simulink model "TBRe19_ECU_SequentialTests"  (R2017b)
settings: Solver=FixedStepDiscrete  StartTime=0.0  StopTime=inf  FixedStep=0.0001  RelTol=1e-3
PostLoadFcn:
  | model_init();
libraries: simulink x28
(part 13 of 22)

== system TBRe19_ECU_SequentialTests/RTDandStateMachine/Pre_Processing_Layer/Pedal_Box ==
  note: Throttle 20 and Brake 10 are arbitrary values (not rules)
  note: Overall Functionality:
      | - All pedal box sensor values are checked to ensure that they are in the correct voltage range
      | - These sensors are then scaled to be between 0-100 %
      | - APPS Implausibility is performed
      | - Brake pedal implausibility is performed
      | - Thresholds for when brake is considered active, and throttle is considered active are set here (used for RTD and Brake Light activation respectively)
  DAL_In : Inport
  APPS and BP Plausibility : Subsystem
  APPS_Implausibility_Check : Subsystem
  BPPS_Implausibility_Check : Subsystem
  Bus Creator : BusCreator  Inputs=12
  Bus Selector : BusSelector  OutputSignals=HAL_Hardwired.Throttle1_Voltage,HAL_Hardwired.Throttle2_Voltage,HAL_Hardwired.Brake_POT,HAL_Hardwired.Brake1_Pressure,HAL_Hardwired.Brake2_Pressure
  Relational Operator : RelationalOperator  OutDataTypeStr=boolean  RndMeth=Simplest
  Relational Operator1 : RelationalOperator  OutDataTypeStr=boolean  RndMeth=Simplest
  Sensor Plausibility : Subsystem
  Terminator : Terminator
  UsbRx : S-Function  FunctionName=NsiUsb_Rx  Parameters=signame,sigtype,resolution,offset,unite,value,is_trigger  SFunctionDeploymentMode=off  EnableBusSupport=off  mask(MUXlink Usb Rx){signame=Brake_Light_Active_Threshold, sigtype=Unsigned Byte, resolution=1, offset=0, unite=%, value=10, is_trigger=off}
      mask prompts: signame "Signal name :"; sigtype "Signal type :"; resolution "Resolution :"; offset "Offset :"; unite "Unit :"; value "Default value :"; is_trigger "Is trigger ?"
      mask help: Receive a frame on the USB Channel.
      mask init:
      | NsiUsb_Rx_InitializationFcn();
      settings: OpenFcn=NsiUsb_Rx_OpenFcn();
      mask Help:
      | eval('block=get_param(gcb, ''RTWdata'');')
      | web([docroot '\toolbox\MUXlink\html\blocks/' block.MUXlink_BlockType '.html'])
      mask Callback signame: NsiUsb_Rx_ApplyFcn(1);
      mask TypeOptions sigtype: Boolean | Signed Byte | Unsigned Byte | Signed Word | Unsigned Word | Signed Double Word | Unsigned Double Word | Single Float | Double Float
      mask Callback sigtype: NsiUsb_Rx_ApplyFcn(2);
      mask Callback resolution: NsiUsb_Rx_ApplyFcn(3);
      mask Callback offset: NsiUsb_Rx_ApplyFcn(4);
      mask Callback unite: NsiUsb_Rx_ApplyFcn(5);
      mask Callback value: NsiUsb_Rx_ApplyFcn(6);
      mask Callback is_trigger: NsiUsb_Rx_ApplyFcn(7);
      mask Display: image(imread('nsi.bmp'));text(0.5, 0.2, 'USB Rx', 'horizontalAlignment', 'center', 'verticalAlignment', 'base');plot([0.05 0.05 0.05 0.05 0.05 0.05 0.05 0.05 0.05 0.05]);port_label('output',1, 'Brake_Light_Active_Threshold');
  UsbRx1 : S-Function  FunctionName=NsiUsb_Rx  Parameters=signame,sigtype,resolution,offset,unite,value,is_trigger  SFunctionDeploymentMode=off  EnableBusSupport=off  mask(MUXlink Usb Rx){signame=Throttle_Active_Threshold, sigtype=Unsigned Byte, resolution=1, offset=0, unite=%, value=5, is_trigger=off}
      mask prompts: signame "Signal name :"; sigtype "Signal type :"; resolution "Resolution :"; offset "Offset :"; unite "Unit :"; value "Default value :"; is_trigger "Is trigger ?"
      mask help: Receive a frame on the USB Channel.
      mask init:
      | NsiUsb_Rx_InitializationFcn();
      settings: OpenFcn=NsiUsb_Rx_OpenFcn();
      mask Help:
      | eval('block=get_param(gcb, ''RTWdata'');')
      | web([docroot '\toolbox\MUXlink\html\blocks/' block.MUXlink_BlockType '.html'])
      mask Callback signame: NsiUsb_Rx_ApplyFcn(1);
      mask TypeOptions sigtype: Boolean | Signed Byte | Unsigned Byte | Signed Word | Unsigned Word | Signed Double Word | Unsigned Double Word | Single Float | Double Float
      mask Callback sigtype: NsiUsb_Rx_ApplyFcn(2);
      mask Callback resolution: NsiUsb_Rx_ApplyFcn(3);
      mask Callback offset: NsiUsb_Rx_ApplyFcn(4);
      mask Callback unite: NsiUsb_Rx_ApplyFcn(5);
      mask Callback value: NsiUsb_Rx_ApplyFcn(6);
      mask Callback is_trigger: NsiUsb_Rx_ApplyFcn(7);
      mask Display: image(imread('nsi.bmp'));text(0.5, 0.2, 'USB Rx', 'horizontalAlignment', 'center', 'verticalAlignment', 'base');plot([0.05 0.05 0.05 0.05 0.05 0.05 0.05 0.05 0.05 0.05]);port_label('output',1, 'Throttle_Active_Threshold');
  Voltage_to_% Conversion : Subsystem
  Pedal_Box_Data : Outport
  wires:
  Bus Creator/1 -> Pedal_Box_Data/1
  DAL_In/1 -> Bus Selector/1
  Voltage_to_% Conversion/1(T1%) -> Bus Creator/2, APPS_Implausibility_Check/1(Throttle1_Per)  "Throttle1_Per"
  Voltage_to_% Conversion/2(T2%) -> Bus Creator/3, APPS_Implausibility_Check/2(Throttle2_Per)  "Throttle2_Per"
  Relational Operator1/1 -> Bus Creator/6  "Throttle_Bool"
  Relational Operator/1 -> Bus Creator/8  "Brake_Bool"
  APPS and BP Plausibility/1(Throttle_%) -> Relational Operator1/1, Bus Creator/5  "Throttle_Percentage"
  APPS and BP Plausibility/2(APPS_BP_Implausibility) -> Bus Creator/7  "APPS_BP_Implausibility"
  APPS_Implausibility_Check/1(APPS_Implausibility) -> Bus Creator/4  "APPS_Implausibility"
  APPS_Implausibility_Check/2(Throttle_%) -> APPS and BP Plausibility/1(Throttle_In)
  Sensor Plausibility/1(Pedal_Sensor_Fail) -> Bus Creator/1  "Pedal_Sensor_Fail"
  Bus Selector/1 -> Sensor Plausibility/1(<Throttle1_Voltage>)  "<Throttle1_Voltage>"
  Bus Selector/2 -> Sensor Plausibility/2(<Throttle2_Voltage>)  "<Throttle2_Voltage>"
  Bus Selector/3 -> Sensor Plausibility/3(<Brake_Voltage>)  "<Brake_POT>"
  Sensor Plausibility/2(TV1_Out) -> Voltage_to_% Conversion/1(Throttle1)
  Sensor Plausibility/3(TV2_Out) -> Voltage_to_% Conversion/2(Throttle2)
  Sensor Plausibility/4(BVPot_Out) -> Voltage_to_% Conversion/3(BrakePOT)
  Bus Selector/4 -> Sensor Plausibility/4(<Brake_Voltage>1)  "<Brake1_Pressure>"
  Bus Selector/5 -> Sensor Plausibility/5(<Brake_Voltage>2)  "<Brake2_Pressure>"
  Sensor Plausibility/5(BV1_Out) -> Voltage_to_% Conversion/4(BrakePress1)
  Sensor Plausibility/6(BV1_Out1) -> Voltage_to_% Conversion/5(BrakePress2)
  BPPS_Implausibility_Check/1(Brake_%) -> Relational Operator/1, Bus Creator/9, APPS and BP Plausibility/2(Brake_%)  "Brake_Percentage"
  BPPS_Implausibility_Check/2(BPPS_Implausibility) -> Bus Creator/10  "BPPS_Implausibility"
  Voltage_to_% Conversion/4(BPr%1) -> Bus Creator/11, BPPS_Implausibility_Check/1(Brake1_Per)  "Brake1_Per"
  Voltage_to_% Conversion/5(BPr%2) -> Bus Creator/12, BPPS_Implausibility_Check/2(Brake2_Per)  "Brake2_Per"
  Voltage_to_% Conversion/3(BPot%) -> Terminator/1  "Brake_%"
  UsbRx/1 -> Relational Operator/2
  UsbRx1/1 -> Relational Operator1/2

== system TBRe19_ECU_SequentialTests/RTDandStateMachine/Vehicle_Functionality_Layer/Vehicle_Operation_Mode ==
  note: Input is zero if error present
  note: NOTE: Check if debounce is needed when coming out of RTD
  note: btnRTD is detected on rising edge
  PrePL_Data : Inport
  Bus Creator : BusCreator  Inputs=5
  Bus Selector1 : BusSelector  OutputSignals=Pedal_Box_Data.Throttle_Bool,Pedal_Box_Data.Brake_Bool,HAL_Data.HAL_Hardwired.btnRTD_Input
  Compare To Constant2 : simulink/Logic and Bit Operations/Compare To Constant  relop=~=  const=0  OutDataTypeStr=boolean
  Operaton_Mode : Stateflow chart  TreatAsAtomicUnit=on
  Rising Edge Detector : Logic  AllPortsSameDT=off  OutDataTypeStr=boolean
  System_Error : Subsystem
  TSS : Subsystem
  Threshold_Level1 : Constant  Value=true  OutDataTypeStr=boolean
  WasZero : Logic  Operator=NOT  AllPortsSameDT=off  OutDataTypeStr=boolean
  prvP2S : Delay  DelayLength=1  InitialCondition=0
  VOM_Data : Outport
  wires:
  Bus Selector1/2 -> Operaton_Mode/2(Brake)  "<Brake_Bool>"
  Compare To Constant2/1 -> Bus Creator/4  "ECU_Ok"
  System_Error/1(System_Error) -> Operaton_Mode/5(Error)
  Operaton_Mode/2(Control_Word) -> Bus Creator/2  "Control_Word"
  Operaton_Mode/1(MCU_NMT_Mode) -> Bus Creator/1  "MCU_NMT_Mode"
  Operaton_Mode/3(State) -> Bus Creator/3, Compare To Constant2/1  "Operation_Mode"
  Bus Creator/1 -> VOM_Data/1  "Vehicle_Operation_Data"
  Bus Selector1/1 -> Operaton_Mode/1(Throttle)  "<Throttle_Bool>"
  PrePL_Data/1 -> Bus Selector1/1, System_Error/1(Errors), TSS/1(PrePL_Data)
  Threshold_Level1/1 -> Operaton_Mode/6(TSS), Bus Creator/5  "TSS"
  WasZero/1 -> Rising Edge Detector/2
  prvP2S/1 -> WasZero/1
  Rising Edge Detector/1 -> Operaton_Mode/3(btnRTD)  "RTD"
  Bus Selector1/3 -> Operaton_Mode/4(btnRTD_Hold), prvP2S/1, Rising Edge Detector/1  "<btnRTD_Input>"

== system TBRe19_ECU_SequentialTests/TSS/Comms_And_Data_Acquisition_Layer/BMS_CAN ==
  note: Overall Functionality:
      | Read CAN messages related to BMS
  Bus Creator4 : BusCreator  Inputs=9
  CanRx6 : S-Function  FunctionName=NsiCan_Rx_Ext  Parameters=data_can,channel,msg_name,ident,ident_type,dlc,signals,is_trigger,is_physical,is_canfd,is_rxgw  SFunctionDeploymentMode=off  EnableBusSupport=off  mask(MUXlink Can Rx){data_can=1;HIGH_SPEED;500Kbps;120 Ohm;C:\Users\TBRe-admin\Documents\Database\TBRe19_DBC_190517.dbc;0;;;0;HIGH_SPEED;500Kbps;120 Ohm;C:\Users\TBRe-admin\Documents\Database\TBRe19_DBC_190517.dbc;0;;;0;HIGH_SPEED;1000Kbps;120 Ohm;D:\TOOLS\MUXLINK\R2011b\MUXlink\misc\BASE_CAN_MUXLAB4.dbc;0;;;0;HIGH_SPEED;500Kbps;120 Ohm;D:\TOOLS\MUXLINK\R2011b\MUXlink\misc\j1939_adapt.dbc;0;;;0;HIGH_SPEED;1000Kbps;No;D:\TOOLS\MUXLINK\R2011b\MUXlink\misc\BASE_CAN_MUXLAB4.dbc;0;;, channel=1, msg_name=BMS_Feedback_1, ident=0x050, ident_type=STD, dlc=7, signals=Instant_Pack_Voltage;1;0;16;1.000000;0.000000;_;Pack_SOC;1;16;16;1.000000;0.000000;_;Pack_Current;1;32;-16;1.000000;64.000000;_;Acc_Fan_Speed;1;48;8;1.000000;0.000000;_, is_trigger=0, is_physical=0, is_canfd=0, is_rxgw=0}
      mask prompts: data_can "data can"; msg_name "msg name"
      mask help: Receive a frame from a CAN channel.
      mask init:
      | NsiCan_Rx_Ext_InitializationFcn();
      settings: OpenFcn=NsiCan_Rx_Ext_OpenFcn();
      mask Help:
      | eval('block=get_param(gcb, ''RTWdata'');')
      | web([docroot '\toolbox\MUXlink\html\blocks/' block.MUXlink_BlockType '.html'])
      mask Callback data_can: NsiCan_Rx_Ext_ApplyFcn(1);
      mask Callback channel: NsiCan_Rx_Ext_ApplyFcn(2);
      mask Callback msg_name: NsiCan_Rx_Ext_ApplyFcn(3);
      mask Callback ident: NsiCan_Rx_Ext_ApplyFcn(4);
      mask Callback ident_type: NsiCan_Rx_Ext_ApplyFcn(5);
      mask Callback dlc: NsiCan_Rx_Ext_ApplyFcn(6);
      mask Callback signals: NsiCan_Rx_Ext_ApplyFcn(7);
      mask Callback is_trigger: NsiCan_Rx_Ext_ApplyFcn(8);
      mask Callback is_physical: NsiCan_Rx_Ext_ApplyFcn(9);
      mask Callback is_canfd: NsiCan_Rx_Ext_ApplyFcn(10);
      mask Callback is_rxgw: NsiCan_Rx_Ext_ApplyFcn(11);
      mask Display: image(imread('nsi.bmp'));text(0.5, 0.3, 'RX_BMS_Feedback_1_CAN1', 'horizontalAlignment', 'center', 'verticalAlignment', 'base');plot([0.05 0.05 0.05 0.05 0.05 0.05 0.05 0.05 0.05 0.05]); port_label('output',1, 'Instant_Pack_Voltage'); port_label('output',2, 'Pack_SOC'); port_label('output',3, 'Pack_Current'); port_label('output',4, 'Acc_Fan_Speed'); port_label('output',5, 'Status');
  CanRx7 : S-Function  FunctionName=NsiCan_Rx_Ext  Parameters=data_can,channel,msg_name,ident,ident_type,dlc,signals,is_trigger,is_physical,is_canfd,is_rxgw  SFunctionDeploymentMode=off  EnableBusSupport=off  mask(MUXlink Can Rx){data_can=1;HIGH_SPEED;500Kbps;No;C:\Users\uvind\OneDrive\Programming\Team Bath Racing Electric\TBRe19_DBC_190621.dbc;0;;;0;HIGH_SPEED;500Kbps;120 Ohm;C:\Users\TBRe-admin\Documents\Database\TBRe19_DBC_190517.dbc;0;;;0;HIGH_SPEED;1000Kbps;120 Ohm;D:\TOOLS\MUXLINK\R2011b\MUXlink\misc\BASE_CAN_MUXLAB4.dbc;0;;;0;HIGH_SPEED;500Kbps;120 Ohm;D:\TOOLS\MUXLINK\R2011b\MUXlink\misc\j1939_adapt.dbc;0;;;0;HIGH_SPEED;1000Kbps;No;D:\TOOLS\MUXLINK\R2011b\MUXlink\misc\BASE_CAN_MUXLAB4.dbc;0;;, channel=1, msg_name=BMS_Feedback_2, ident=0x051, ident_type=STD, dlc=8, signals=Avg_Cell_Voltage;1;32;16;1.000000;0.000000;_;High_Cell_Voltage;1;16;16;1.000000;0.000000;_;High_Cell_ID;1;56;8;1.000000;0.000000;_;Low_Cell_Voltage;1;0;16;1.000000;0.000000;_;Low_Cell_ID;1;48;8;1.000000;0.000000;_, is_trigger=0, is_physical=0, is_canfd=0, is_rxgw=0}
      mask prompts: data_can "data can"; msg_name "msg name"
      mask help: Receive a frame from a CAN channel.
      mask init:
      | NsiCan_Rx_Ext_InitializationFcn();
      settings: OpenFcn=NsiCan_Rx_Ext_OpenFcn();
      mask Help:
      | eval('block=get_param(gcb, ''RTWdata'');')
      | web([docroot '\toolbox\MUXlink\html\blocks/' block.MUXlink_BlockType '.html'])
      mask Callback data_can: NsiCan_Rx_Ext_ApplyFcn(1);
      mask Callback channel: NsiCan_Rx_Ext_ApplyFcn(2);
      mask Callback msg_name: NsiCan_Rx_Ext_ApplyFcn(3);
      mask Callback ident: NsiCan_Rx_Ext_ApplyFcn(4);
      mask Callback ident_type: NsiCan_Rx_Ext_ApplyFcn(5);
      mask Callback dlc: NsiCan_Rx_Ext_ApplyFcn(6);
      mask Callback signals: NsiCan_Rx_Ext_ApplyFcn(7);
      mask Callback is_trigger: NsiCan_Rx_Ext_ApplyFcn(8);
      mask Callback is_physical: NsiCan_Rx_Ext_ApplyFcn(9);
      mask Callback is_canfd: NsiCan_Rx_Ext_ApplyFcn(10);
      mask Callback is_rxgw: NsiCan_Rx_Ext_ApplyFcn(11);
      mask Display: image(imread('nsi.bmp'));text(0.5, 0.3, 'RX_BMS_Feedback_2_CAN1', 'horizontalAlignment', 'center', 'verticalAlignment', 'base');plot([0.05 0.05 0.05 0.05 0.05 0.05 0.05 0.05 0.05 0.05]); port_label('output',1, 'Avg_Cell_Voltage'); port_label('output',2, 'High_Cell_Voltage'); port_label('output',3, 'High_Cell_ID'); port_label('output',4, 'Low_Cell_Voltage'); port_label('output',5, 'Low_Cell_ID'); port_label('output',6, 'Status');
  BMS_Data : Outport
  wires:
  CanRx6/5 -> ?
  CanRx7/6 -> ?
  CanRx6/3 -> Bus Creator4/3  "Pack_Current"
  CanRx6/1 -> Bus Creator4/1  "Instant_Pack_Voltage"
  CanRx7/3 -> Bus Creator4/7  "High_Cell_ID"
  CanRx6/4 -> Bus Creator4/4  "Acc_Fan_Speed"
  CanRx7/1 -> Bus Creator4/5  "Abg_Cell_Voltage"
  Bus Creator4/1 -> BMS_Data/1  "BMS_Data"
  CanRx7/5 -> Bus Creator4/9  "Low_Cell_ID"
  CanRx7/2 -> Bus Creator4/6  "High_Cell_Voltage"
  CanRx7/4 -> Bus Creator4/8  "Low_Cell_Voltage"
  CanRx6/2 -> Bus Creator4/2  "Pack_SOC"

== system TBRe19_ECU_SequentialTests/TSS/Comms_And_Data_Acquisition_Layer/Hardwired_Inputs_2019 ==
  note: Action:
      | Put the inputs into bus and generate output
  note: Overall Functionality:
      | Get inputs from the physical input pins
  AIRs : Subsystem
  BMS : Subsystem
  Bus Creator : BusCreator  Inputs=18
  Buttons : Subsystem
  FrequentialInput1 : S-Function  FunctionName=NsiIo_FrequencyInput  Parameters=channel,max_freq,is_digital_input,DutyCycle,MUXlabType  SFunctionDeploymentMode=off  EnableBusSupport=off  mask(MUXlink I/O Frequential Input){channel=3, max_freq=10KHZ, is_digital_input=off, DutyCycle=off, MUXlabType=0}
      mask prompts: max_freq "Max Frequency"; is_digital_input "Used as Digital Input"; DutyCycle "Duty Cycle"; MUXlabType "MUXlab Type"
      mask help: Read Frequency from I/O Frequential Input.
      mask init:
      | NsiIo_FrequencyInput_InitializationFcn();
      settings: OpenFcn=NsiIo_FrequencyInput_OpenFcn();
      mask Help:
      | eval('block=get_param(gcb, ''RTWdata'');')
      | web([docroot '\toolbox\MUXlink\html\blocks/' block.MUXlink_BlockType '.html'])
      mask Callback channel: NsiIo_FrequencyInput_ApplyFcn(1);
      mask TypeOptions max_freq: 10KHZ | 100KHZ
      mask Callback max_freq: NsiIo_FrequencyInput_ApplyFcn(2);
      mask Callback is_digital_input: NsiIo_FrequencyInput_ApplyFcn(3);
      mask Callback DutyCycle: NsiIo_FrequencyInput_ApplyFcn(4);
      mask Display: image(imread('nsi.bmp'));text(0.5, 0.2, 'FrequencyInput_3  10KHZ', 'horizontalAlignment', 'center', 'verticalAlignment', 'base');plot([0.05 0.05 0.05 0.05 0.05 0.05 0.05 0.05 0.05 0.05]);port_label('output', 1, 'Freq C3');
  Pedal_Box : Subsystem
  VBat : S-Function  FunctionName=NsiIo_Vbat  SFunctionDeploymentMode=off  EnableBusSupport=off  mask(MUXlink I/O VBat){}
      mask help: Battery Voltage
      mask init:
      | NsiIo_Vbat_InitializationFcn();
      settings: OpenFcn=NsiIo_Vbat_OpenFcn();
      mask Help:
      | eval('block=get_param(gcb, ''RTWdata'');')
      | web([docroot '\toolbox\MUXlink\html\blocks/' block.MUXlink_BlockType '.html'])
      mask Display: image(imread('nsi.bmp'));text(0.5, 0.2, 'I/O VBat', 'horizontalAlignment', 'center', 'verticalAlignment', 'base');plot([0.05 0.05 0.05 0.05 0.05 0.05 0.05 0.05 0.05 0.05]);port_label('output', 1, 'Voltage');
  Hardwired_Inputs : Outport
  wires:
  VBat/1 -> Bus Creator/12  "LV_Battery_Voltage"
  FrequentialInput1/1 -> Bus Creator/13  "Fan_Freq"
  Bus Creator/1 -> Hardwired_Inputs/1
  Pedal_Box/1(Throttle1_Voltage) -> Bus Creator/1
  Pedal_Box/2(Throttle2_Voltage) -> Bus Creator/2
  Pedal_Box/3(Brake_Voltage) -> Bus Creator/3
  Buttons/1(btnRTD_Input) -> Bus Creator/6
  Buttons/2(btnX_Input) -> Bus Creator/7
  Buttons/3(btnY_Input) -> Bus Creator/8
  AIRs/1(AIRLow) -> Bus Creator/14
  AIRs/2(AIRHigh) -> Bus Creator/15
  Pedal_Box/4(Brake1_Pressure) -> Bus Creator/4
  Pedal_Box/5(Brake2_Pressure) -> Bus Creator/5
  Buttons/4(btnZ_Input) -> Bus Creator/9
  Buttons/5(btnPumpFan_Input) -> Bus Creator/10
  Buttons/6(btnAccyFan_Input) -> Bus Creator/11
  BMS/1(BMS_Multi1) -> Bus Creator/16
  BMS/2(BMS_Multi2) -> Bus Creator/17
  BMS/3(BMS_ChargeEnable) -> Bus Creator/18

== system TBRe19_ECU_SequentialTests/TSS/Comms_And_Data_Acquisition_Layer/MCU_CAN ==
  note: Overall Functionality:
      | Read CAN messages related to motor control unit (MCU)
  Bus Creator1 : BusCreator  Inputs=4
  CanRx1 : S-Function  FunctionName=NsiCan_Rx_J1939_Ext  Parameters=data_can,channel,msg_name,ident,ident_type,dlc,signals,is_trigger,is_SA_Masked,is_TA_Masked,is_physical,is_canfd  SFunctionDeploymentMode=off  EnableBusSupport=off  mask(MUXlink Can Rx){data_can=1;HIGH_SPEED;500Kbps;No;C:\Users\TBRe-admin\Documents\Database\TBRe19_DBC_190617.dbc;0;;;0;HIGH_SPEED;500Kbps;120 Ohm;C:\Users\TBRe-admin\Documents\Database\TBRe19_DBC_190517.dbc;0;;;0;HIGH_SPEED;1000Kbps;120 Ohm;D:\TOOLS\MUXLINK\R2011b\MUXlink\misc\BASE_CAN_MUXLAB4.dbc;0;;;0;HIGH_SPEED;500Kbps;120 Ohm;D:\TOOLS\MUXLINK\R2011b\MUXlink\misc\j1939_adapt.dbc;0;;;0;HIGH_SPEED;1000Kbps;No;D:\TOOLS\MUXLINK\R2011b\MUXlink\misc\BASE_CAN_MUXLAB4.dbc;0;;, channel=1, msg_name=HS3_Temperature_Feedback, ident=0x191AFF71, ident_type=XTD, dlc=8, signals=DC_Link_Voltage;1;32;-16;0.062500;0.000000;V;MotorTemperature;1;16;-16;1.000000;0.000000;C, is_trigger=0, is_physical=0, is_canfd=0, is_SA_Masked=1, is_TA_Masked=0}
      mask prompts: data_can "data can"; msg_name "msg name"; is_SA_Masked "J1939 SA filtering"; is_TA_Masked "J1939 TA filtering"
      mask help: Receive a frame from a CAN channel.
      mask init:
      | NsiCan_Rx_J1939_Ext_InitializationFcn();
      settings: OpenFcn=NsiCan_Rx_J1939_Ext_OpenFcn();
      mask Help:
      | eval('block=get_param(gcb, ''RTWdata'');')
      | web([docroot '\toolbox\MUXlink\html\blocks/' block.MUXlink_BlockType '.html'])
      mask Callback data_can: NsiCan_Rx_J1939_Ext_ApplyFcn(1);
      mask Callback channel: NsiCan_Rx_J1939_Ext_ApplyFcn(2);
      mask Callback msg_name: NsiCan_Rx_J1939_Ext_ApplyFcn(3);
      mask Callback ident: NsiCan_Rx_J1939_Ext_ApplyFcn(4);
      mask Callback ident_type: NsiCan_Rx_J1939_Ext_ApplyFcn(5);
      mask Callback dlc: NsiCan_Rx_J1939_Ext_ApplyFcn(6);
      mask Callback signals: NsiCan_Rx_J1939_Ext_ApplyFcn(7);
      mask Callback is_trigger: NsiCan_Rx_J1939_Ext_ApplyFcn(8);
      mask Callback is_physical: NsiCan_Rx_J1939_Ext_ApplyFcn(9);
      mask Callback is_canfd: NsiCan_Rx_J1939_Ext_ApplyFcn(10);
      mask Callback is_SA_Masked: NsiCan_Rx_J1939_Ext_ApplyFcn(11);
      mask Callback is_TA_Masked: NsiCan_Rx_J1939_Ext_ApplyFcn(12);
      mask Display: image(imread('nsi.bmp'));text(0.5, 0.3, 'J1939_PGN  HS3_Temperature_Feedbackchannel CAN1', 'horizontalAlignment', 'center', 'verticalAlignment', 'base');plot([0.05 0.05 0.05 0.05 0.05 0.05 0.05 0.05 0.05 0.05]); port_label('output',1, 'DC_Link_Voltage'); port_label('output',2, 'MotorTemperature'); port_label('output',3, 'Status');
  CanRx2 : S-Function  FunctionName=NsiCan_Rx_J1939_Ext  Parameters=data_can,channel,msg_name,ident,ident_type,dlc,signals,is_trigger,is_SA_Masked,is_TA_Masked,is_physical,is_canfd  SFunctionDeploymentMode=off  EnableBusSupport=off  mask(MUXlink Can Rx){data_can=1;HIGH_SPEED;500Kbps;No;C:\Users\TBRe-admin\Documents\Database\TBRe19_DBC_190617.dbc;0;;;0;HIGH_SPEED;500Kbps;120 Ohm;C:\Users\TBRe-admin\Documents\Database\TBRe19_DBC_190517.dbc;0;;;0;HIGH_SPEED;1000Kbps;120 Ohm;D:\TOOLS\MUXLINK\R2011b\MUXlink\misc\BASE_CAN_MUXLAB4.dbc;0;;;0;HIGH_SPEED;500Kbps;120 Ohm;D:\TOOLS\MUXLINK\R2011b\MUXlink\misc\j1939_adapt.dbc;0;;;0;HIGH_SPEED;1000Kbps;No;D:\TOOLS\MUXLINK\R2011b\MUXlink\misc\BASE_CAN_MUXLAB4.dbc;0;;, channel=1, msg_name=HD4_Debug_Temperatures_B, ident=0x192BFF71, ident_type=XTD, dlc=8, signals=Debug_Temps_Heatsink;1;24;8;1.000000;0.000000;degC, is_trigger=0, is_physical=0, is_canfd=0, is_SA_Masked=1, is_TA_Masked=0}
      mask prompts: data_can "data can"; msg_name "msg name"; is_SA_Masked "J1939 SA filtering"; is_TA_Masked "J1939 TA filtering"
      mask help: Receive a frame from a CAN channel.
      mask init:
      | NsiCan_Rx_J1939_Ext_InitializationFcn();
      settings: OpenFcn=NsiCan_Rx_J1939_Ext_OpenFcn();
      mask Help:
      | eval('block=get_param(gcb, ''RTWdata'');')
      | web([docroot '\toolbox\MUXlink\html\blocks/' block.MUXlink_BlockType '.html'])
      mask Callback data_can: NsiCan_Rx_J1939_Ext_ApplyFcn(1);
      mask Callback channel: NsiCan_Rx_J1939_Ext_ApplyFcn(2);
      mask Callback msg_name: NsiCan_Rx_J1939_Ext_ApplyFcn(3);
      mask Callback ident: NsiCan_Rx_J1939_Ext_ApplyFcn(4);
      mask Callback ident_type: NsiCan_Rx_J1939_Ext_ApplyFcn(5);
      mask Callback dlc: NsiCan_Rx_J1939_Ext_ApplyFcn(6);
      mask Callback signals: NsiCan_Rx_J1939_Ext_ApplyFcn(7);
      mask Callback is_trigger: NsiCan_Rx_J1939_Ext_ApplyFcn(8);
      mask Callback is_physical: NsiCan_Rx_J1939_Ext_ApplyFcn(9);
      mask Callback is_canfd: NsiCan_Rx_J1939_Ext_ApplyFcn(10);
      mask Callback is_SA_Masked: NsiCan_Rx_J1939_Ext_ApplyFcn(11);
      mask Callback is_TA_Masked: NsiCan_Rx_J1939_Ext_ApplyFcn(12);
      mask Display: image(imread('nsi.bmp'));text(0.5, 0.3, 'J1939_PGN  HD4_Debug_Temperatures_Bchannel CAN1', 'horizontalAlignment', 'center', 'verticalAlignment', 'base');plot([0.05 0.05 0.05 0.05 0.05 0.05 0.05 0.05 0.05 0.05]); port_label('output',1, 'Debug_Temps_Heatsink'); port_label('output',2, 'Status');
  CanRx3 : S-Function  FunctionName=NsiCan_Rx_J1939_Ext  Parameters=data_can,channel,msg_name,ident,ident_type,dlc,signals,is_trigger,is_SA_Masked,is_TA_Masked,is_physical,is_canfd  SFunctionDeploymentMode=off  EnableBusSupport=off  mask(MUXlink Can Rx){data_can=1;HIGH_SPEED;500Kbps;No;C:\Users\TBRe-admin\Documents\Database\TBRe19_DBC_190617.dbc;0;;;0;HIGH_SPEED;500Kbps;120 Ohm;C:\Users\TBRe-admin\Documents\Database\TBRe19_DBC_190517.dbc;0;;;0;HIGH_SPEED;1000Kbps;120 Ohm;D:\TOOLS\MUXLINK\R2011b\MUXlink\misc\BASE_CAN_MUXLAB4.dbc;0;;;0;HIGH_SPEED;500Kbps;120 Ohm;D:\TOOLS\MUXLINK\R2011b\MUXlink\misc\j1939_adapt.dbc;0;;;0;HIGH_SPEED;1000Kbps;No;D:\TOOLS\MUXLINK\R2011b\MUXlink\misc\BASE_CAN_MUXLAB4.dbc;0;;, channel=1, msg_name=HS1_Torque_Feedback, ident=0x1918FF71, ident_type=XTD, dlc=8, signals=Speed_Measured;1;16;-16;1.000000;0.000000;RPM, is_trigger=0, is_physical=0, is_canfd=0, is_SA_Masked=1, is_TA_Masked=0}
      mask prompts: data_can "data can"; msg_name "msg name"; is_SA_Masked "J1939 SA filtering"; is_TA_Masked "J1939 TA filtering"
      mask help: Receive a frame from a CAN channel.
      mask init:
      | NsiCan_Rx_J1939_Ext_InitializationFcn();
      settings: OpenFcn=NsiCan_Rx_J1939_Ext_OpenFcn();
      mask Help:
      | eval('block=get_param(gcb, ''RTWdata'');')
      | web([docroot '\toolbox\MUXlink\html\blocks/' block.MUXlink_BlockType '.html'])
      mask Callback data_can: NsiCan_Rx_J1939_Ext_ApplyFcn(1);
      mask Callback channel: NsiCan_Rx_J1939_Ext_ApplyFcn(2);
      mask Callback msg_name: NsiCan_Rx_J1939_Ext_ApplyFcn(3);
      mask Callback ident: NsiCan_Rx_J1939_Ext_ApplyFcn(4);
      mask Callback ident_type: NsiCan_Rx_J1939_Ext_ApplyFcn(5);
      mask Callback dlc: NsiCan_Rx_J1939_Ext_ApplyFcn(6);
      mask Callback signals: NsiCan_Rx_J1939_Ext_ApplyFcn(7);
      mask Callback is_trigger: NsiCan_Rx_J1939_Ext_ApplyFcn(8);
      mask Callback is_physical: NsiCan_Rx_J1939_Ext_ApplyFcn(9);
      mask Callback is_canfd: NsiCan_Rx_J1939_Ext_ApplyFcn(10);
      mask Callback is_SA_Masked: NsiCan_Rx_J1939_Ext_ApplyFcn(11);
      mask Callback is_TA_Masked: NsiCan_Rx_J1939_Ext_ApplyFcn(12);
      mask Display: image(imread('nsi.bmp'));text(0.5, 0.3, 'J1939_PGN  HS1_Torque_Feedbackchannel CAN1', 'horizontalAlignment', 'center', 'verticalAlignment', 'base');plot([0.05 0.05 0.05 0.05 0.05 0.05 0.05 0.05 0.05 0.05]); port_label('output',1, 'Speed_Measured'); port_label('output',2, 'Status');
  HAL_MCU : Outport
  wires:
  Bus Creator1/1 -> HAL_MCU/1  "HAL_MCU"
  CanRx1/1 -> Bus Creator1/1  "MCU_Voltage"
  CanRx1/2 -> Bus Creator1/2  "Motor_Temp"
  CanRx2/1 -> Bus Creator1/3  "MCU_Temp"
  CanRx3/1 -> Bus Creator1/4  "Motor_Speed"

== system TBRe19_ECU_SequentialTests/TSS/Comms_And_Data_Acquisition_Layer/SENSOR_CAN ==
  note: Overall Functionality:
      | Read CAN messages related to vehicle sensors
  Bus Creator3 : BusCreator  Inputs=9
  CanRx1 : S-Function  FunctionName=NsiCan_Rx_Ext  Parameters=data_can,channel,msg_name,ident,ident_type,dlc,signals,is_trigger,is_physical,is_canfd,is_rxgw  SFunctionDeploymentMode=off  EnableBusSupport=off  mask(MUXlink Can Rx){data_can=1;HIGH_SPEED;500Kbps;No;C:\Users\TBRe-admin\Documents\Database\TBRe19_DBC_190617.dbc;0;;;0;HIGH_SPEED;500Kbps;120 Ohm;C:\Users\TBRe-admin\Documents\Database\TBRe19_DBC_190517.dbc;0;;;0;HIGH_SPEED;1000Kbps;120 Ohm;D:\TOOLS\MUXLINK\R2011b\MUXlink\misc\BASE_CAN_MUXLAB4.dbc;0;;;0;HIGH_SPEED;500Kbps;120 Ohm;D:\TOOLS\MUXLINK\R2011b\MUXlink\misc\j1939_adapt.dbc;0;;;0;HIGH_SPEED;1000Kbps;No;D:\TOOLS\MUXLINK\R2011b\MUXlink\misc\BASE_CAN_MUXLAB4.dbc;0;;, channel=1, msg_name=Front_Wheel_Speeds, ident=0x502, ident_type=STD, dlc=6, signals=Front_Left_Wheel_Speed;1;16;16;0.100000;0.000000;rpm;Front_Right_Wheel_Speed;1;0;16;0.100000;0.000000;rpm;Vehicle_Speed;1;32;16;0.010000;0.000000;_, is_trigger=0, is_physical=0, is_canfd=0, is_rxgw=0}
      mask prompts: data_can "data can"; msg_name "msg name"
      mask help: Receive a frame from a CAN channel.
      mask init:
      | NsiCan_Rx_Ext_InitializationFcn();
      settings: OpenFcn=NsiCan_Rx_Ext_OpenFcn();
      mask Help:
      | eval('block=get_param(gcb, ''RTWdata'');')
      | web([docroot '\toolbox\MUXlink\html\blocks/' block.MUXlink_BlockType '.html'])
      mask Callback data_can: NsiCan_Rx_Ext_ApplyFcn(1);
      mask Callback channel: NsiCan_Rx_Ext_ApplyFcn(2);
      mask Callback msg_name: NsiCan_Rx_Ext_ApplyFcn(3);
      mask Callback ident: NsiCan_Rx_Ext_ApplyFcn(4);
      mask Callback ident_type: NsiCan_Rx_Ext_ApplyFcn(5);
      mask Callback dlc: NsiCan_Rx_Ext_ApplyFcn(6);
      mask Callback signals: NsiCan_Rx_Ext_ApplyFcn(7);
      mask Callback is_trigger: NsiCan_Rx_Ext_ApplyFcn(8);
      mask Callback is_physical: NsiCan_Rx_Ext_ApplyFcn(9);
      mask Callback is_canfd: NsiCan_Rx_Ext_ApplyFcn(10);
      mask Callback is_rxgw: NsiCan_Rx_Ext_ApplyFcn(11);
      mask Display: image(imread('nsi.bmp'));text(0.5, 0.3, 'RX_Front_Wheel_Speeds_CAN1', 'horizontalAlignment', 'center', 'verticalAlignment', 'base');plot([0.05 0.05 0.05 0.05 0.05 0.05 0.05 0.05 0.05 0.05]); port_label('output',1, 'Front_Left_Wheel_Speed'); port_label('output',2, 'Front_Right_Wheel_Speed'); port_label('output',3, 'Vehicle_Speed'); port_label('output',4, 'Status');
  CanRx2 : S-Function  FunctionName=NsiCan_Rx_Ext  Parameters=data_can,channel,msg_name,ident,ident_type,dlc,signals,is_trigger,is_physical,is_canfd,is_rxgw  SFunctionDeploymentMode=off  EnableBusSupport=off  mask(MUXlink Can Rx){data_can=1;HIGH_SPEED;500Kbps;No;C:\Users\TBRe-admin\Documents\Database\TBRe19_DBC_190617.dbc;0;;;0;HIGH_SPEED;500Kbps;120 Ohm;C:\Users\TBRe-admin\Documents\Database\TBRe19_DBC_190517.dbc;0;;;0;HIGH_SPEED;1000Kbps;120 Ohm;D:\TOOLS\MUXLINK\R2011b\MUXlink\misc\BASE_CAN_MUXLAB4.dbc;0;;;0;HIGH_SPEED;500Kbps;120 Ohm;D:\TOOLS\MUXLINK\R2011b\MUXlink\misc\j1939_adapt.dbc;0;;;0;HIGH_SPEED;1000Kbps;No;D:\TOOLS\MUXLINK\R2011b\MUXlink\misc\BASE_CAN_MUXLAB4.dbc;0;;, channel=1, msg_name=Rear_Wheel_Speed, ident=0x501, ident_type=STD, dlc=6, signals=Rear_Left_Wheel_Speed;1;16;16;0.100000;0.000000;rpm;Rear_Right_Wheel_Speed;1;0;16;0.100000;0.000000;rpm;Rear_Wheel_Speed;1;32;16;0.010000;0.000000;km/h, is_trigger=0, is_physical=0, is_canfd=0, is_rxgw=0}
      mask prompts: data_can "data can"; msg_name "msg name"
      mask help: Receive a frame from a CAN channel.
      mask init:
      | NsiCan_Rx_Ext_InitializationFcn();
      settings: OpenFcn=NsiCan_Rx_Ext_OpenFcn();
      mask Help:
      | eval('block=get_param(gcb, ''RTWdata'');')
      | web([docroot '\toolbox\MUXlink\html\blocks/' block.MUXlink_BlockType '.html'])
      mask Callback data_can: NsiCan_Rx_Ext_ApplyFcn(1);
      mask Callback channel: NsiCan_Rx_Ext_ApplyFcn(2);
      mask Callback msg_name: NsiCan_Rx_Ext_ApplyFcn(3);
      mask Callback ident: NsiCan_Rx_Ext_ApplyFcn(4);
      mask Callback ident_type: NsiCan_Rx_Ext_ApplyFcn(5);
      mask Callback dlc: NsiCan_Rx_Ext_ApplyFcn(6);
      mask Callback signals: NsiCan_Rx_Ext_ApplyFcn(7);
      mask Callback is_trigger: NsiCan_Rx_Ext_ApplyFcn(8);
      mask Callback is_physical: NsiCan_Rx_Ext_ApplyFcn(9);
      mask Callback is_canfd: NsiCan_Rx_Ext_ApplyFcn(10);
      mask Callback is_rxgw: NsiCan_Rx_Ext_ApplyFcn(11);
      mask Display: image(imread('nsi.bmp'));text(0.5, 0.3, 'RX_Rear_Wheel_Speed_CAN1', 'horizontalAlignment', 'center', 'verticalAlignment', 'base');plot([0.05 0.05 0.05 0.05 0.05 0.05 0.05 0.05 0.05 0.05]); port_label('output',1, 'Rear_Left_Wheel_Speed'); port_label('output',2, 'Rear_Right_Wheel_Speed'); port_label('output',3, 'Rear_Wheel_Speed'); port_label('output',4, 'Status');
  CanRx5 : S-Function  FunctionName=NsiCan_Rx_Ext  Parameters=data_can,channel,msg_name,ident,ident_type,dlc,signals,is_trigger,is_physical,is_canfd,is_rxgw  SFunctionDeploymentMode=off  EnableBusSupport=off  mask(MUXlink Can Rx){data_can=1;HIGH_SPEED;500Kbps;No;C:\Users\TBRe-admin\Documents\Database\TBRe19_DBC_190617.dbc;0;;;0;HIGH_SPEED;500Kbps;120 Ohm;C:\Users\TBRe-admin\Documents\Database\TBRe19_DBC_190517.dbc;0;;;0;HIGH_SPEED;1000Kbps;120 Ohm;D:\TOOLS\MUXLINK\R2011b\MUXlink\misc\BASE_CAN_MUXLAB4.dbc;0;;;0;HIGH_SPEED;500Kbps;120 Ohm;D:\TOOLS\MUXLINK\R2011b\MUXlink\misc\j1939_adapt.dbc;0;;;0;HIGH_SPEED;1000Kbps;No;D:\TOOLS\MUXLINK\R2011b\MUXlink\misc\BASE_CAN_MUXLAB4.dbc;0;;, channel=1, msg_name=SteeringWheelSensor, ident=0x234, ident_type=STD, dlc=5, signals=Acc_Angle;1;0;-16;0.100000;0.000000;Degrees, is_trigger=0, is_physical=0, is_canfd=0, is_rxgw=0}
      mask prompts: data_can "data can"; msg_name "msg name"
      mask help: Receive a frame from a CAN channel.
      mask init:
      | NsiCan_Rx_Ext_InitializationFcn();
      settings: OpenFcn=NsiCan_Rx_Ext_OpenFcn();
      mask Help:
      | eval('block=get_param(gcb, ''RTWdata'');')
      | web([docroot '\toolbox\MUXlink\html\blocks/' block.MUXlink_BlockType '.html'])
      mask Callback data_can: NsiCan_Rx_Ext_ApplyFcn(1);
      mask Callback channel: NsiCan_Rx_Ext_ApplyFcn(2);
      mask Callback msg_name: NsiCan_Rx_Ext_ApplyFcn(3);
      mask Callback ident: NsiCan_Rx_Ext_ApplyFcn(4);
      mask Callback ident_type: NsiCan_Rx_Ext_ApplyFcn(5);
      mask Callback dlc: NsiCan_Rx_Ext_ApplyFcn(6);
      mask Callback signals: NsiCan_Rx_Ext_ApplyFcn(7);
      mask Callback is_trigger: NsiCan_Rx_Ext_ApplyFcn(8);
      mask Callback is_physical: NsiCan_Rx_Ext_ApplyFcn(9);
      mask Callback is_canfd: NsiCan_Rx_Ext_ApplyFcn(10);
      mask Callback is_rxgw: NsiCan_Rx_Ext_ApplyFcn(11);
      mask Display: image(imread('nsi.bmp'));text(0.5, 0.3, 'RX_SteeringWheelSensor_CAN1', 'horizontalAlignment', 'center', 'verticalAlignment', 'base');plot([0.05 0.05 0.05 0.05 0.05 0.05 0.05 0.05 0.05 0.05]); port_label('output',1, 'Acc_Angle'); port_label('output',2, 'Status');
  CanRx8 : S-Function  FunctionName=NsiCan_Rx_Ext  Parameters=data_can,channel,msg_name,ident,ident_type,dlc,signals,is_trigger,is_physical,is_canfd,is_rxgw  SFunctionDeploymentMode=off  EnableBusSupport=off  mask(MUXlink Can Rx){data_can=1;HIGH_SPEED;500Kbps;No;C:\Users\TBRe-admin\Documents\Database\TBRe19_DBC_190617.dbc;0;;;0;HIGH_SPEED;500Kbps;120 Ohm;C:\Users\TBRe-admin\Documents\Database\TBRe19_DBC_190517.dbc;0;;;0;HIGH_SPEED;1000Kbps;120 Ohm;D:\TOOLS\MUXLINK\R2011b\MUXlink\misc\BASE_CAN_MUXLAB4.dbc;0;;;0;HIGH_SPEED;500Kbps;120 Ohm;D:\TOOLS\MUXLINK\R2011b\MUXlink\misc\j1939_adapt.dbc;0;;;0;HIGH_SPEED;1000Kbps;No;D:\TOOLS\MUXLINK\R2011b\MUXlink\misc\BASE_CAN_MUXLAB4.dbc;0;;, channel=1, msg_name=AccelerometerY, ident=0x174, ident_type=STD, dlc=8, signals=Acc_Yaw;1;0;16;0.005000;0.000000;_, is_trigger=0, is_physical=0, is_canfd=0, is_rxgw=0}
      mask prompts: data_can "data can"; msg_name "msg name"
      mask help: Receive a frame from a CAN channel.
      mask init:
      | NsiCan_Rx_Ext_InitializationFcn();
      settings: OpenFcn=NsiCan_Rx_Ext_OpenFcn();
      mask Help:
      | eval('block=get_param(gcb, ''RTWdata'');')
      | web([docroot '\toolbox\MUXlink\html\blocks/' block.MUXlink_BlockType '.html'])
      mask Callback data_can: NsiCan_Rx_Ext_ApplyFcn(1);
      mask Callback channel: NsiCan_Rx_Ext_ApplyFcn(2);
      mask Callback msg_name: NsiCan_Rx_Ext_ApplyFcn(3);
      mask Callback ident: NsiCan_Rx_Ext_ApplyFcn(4);
      mask Callback ident_type: NsiCan_Rx_Ext_ApplyFcn(5);
      mask Callback dlc: NsiCan_Rx_Ext_ApplyFcn(6);
      mask Callback signals: NsiCan_Rx_Ext_ApplyFcn(7);
      mask Callback is_trigger: NsiCan_Rx_Ext_ApplyFcn(8);
      mask Callback is_physical: NsiCan_Rx_Ext_ApplyFcn(9);
      mask Callback is_canfd: NsiCan_Rx_Ext_ApplyFcn(10);
      mask Callback is_rxgw: NsiCan_Rx_Ext_ApplyFcn(11);
      mask Display: image(imread('nsi.bmp'));text(0.5, 0.3, 'RX_AccelerometerY_CAN1', 'horizontalAlignment', 'center', 'verticalAlignment', 'base');plot([0.05 0.05 0.05 0.05 0.05 0.05 0.05 0.05 0.05 0.05]); port_label('output',1, 'Acc_Yaw'); port_label('output',2, 'Status');
  CanRx9 : S-Function  FunctionName=NsiCan_Rx_Ext  Parameters=data_can,channel,msg_name,ident,ident_type,dlc,signals,is_trigger,is_physical,is_canfd,is_rxgw  SFunctionDeploymentMode=off  EnableBusSupport=off  mask(MUXlink Can Rx){data_can=1;HIGH_SPEED;500Kbps;No;C:\Users\TBRe-admin\Documents\Database\TBRe19_DBC_190620.dbc;0;;;0;HIGH_SPEED;500Kbps;120 Ohm;C:\Users\TBRe-admin\Documents\Database\TBRe19_DBC_190517.dbc;0;;;0;HIGH_SPEED;1000Kbps;120 Ohm;D:\TOOLS\MUXLINK\R2011b\MUXlink\misc\BASE_CAN_MUXLAB4.dbc;0;;;0;HIGH_SPEED;500Kbps;120 Ohm;D:\TOOLS\MUXLINK\R2011b\MUXlink\misc\j1939_adapt.dbc;0;;;0;HIGH_SPEED;1000Kbps;No;D:\TOOLS\MUXLINK\R2011b\MUXlink\misc\BASE_CAN_MUXLAB4.dbc;0;;, channel=1, msg_name=Shutdown_Data, ident=0x705, ident_type=STD, dlc=3, signals=Fault_CarShutdown;1;0;1;1.000000;0.000000;_, is_trigger=0, is_physical=0, is_canfd=0, is_rxgw=0}
      mask prompts: data_can "data can"; msg_name "msg name"
      mask help: Receive a frame from a CAN channel.
      mask init:
      | NsiCan_Rx_Ext_InitializationFcn();
      settings: OpenFcn=NsiCan_Rx_Ext_OpenFcn();
      mask Help:
      | eval('block=get_param(gcb, ''RTWdata'');')
      | web([docroot '\toolbox\MUXlink\html\blocks/' block.MUXlink_BlockType '.html'])
      mask Callback data_can: NsiCan_Rx_Ext_ApplyFcn(1);
      mask Callback channel: NsiCan_Rx_Ext_ApplyFcn(2);
      mask Callback msg_name: NsiCan_Rx_Ext_ApplyFcn(3);
      mask Callback ident: NsiCan_Rx_Ext_ApplyFcn(4);
      mask Callback ident_type: NsiCan_Rx_Ext_ApplyFcn(5);
      mask Callback dlc: NsiCan_Rx_Ext_ApplyFcn(6);
      mask Callback signals: NsiCan_Rx_Ext_ApplyFcn(7);
      mask Callback is_trigger: NsiCan_Rx_Ext_ApplyFcn(8);
      mask Callback is_physical: NsiCan_Rx_Ext_ApplyFcn(9);
      mask Callback is_canfd: NsiCan_Rx_Ext_ApplyFcn(10);
      mask Callback is_rxgw: NsiCan_Rx_Ext_ApplyFcn(11);
      mask Display: image(imread('nsi.bmp'));text(0.5, 0.3, 'RX_Shutdown_Data_CAN1', 'horizontalAlignment', 'center', 'verticalAlignment', 'base');plot([0.05 0.05 0.05 0.05 0.05 0.05 0.05 0.05 0.05 0.05]); port_label('output',1, 'Fault_CarShutdown'); port_label('output',2, 'Status');
  Sensor_Data : Outport
  wires:
  CanRx5/2 -> ?
  CanRx1/4 -> ?
  CanRx2/4 -> ?
  CanRx8/2 -> ?
  CanRx9/2 -> ?
  CanRx9/1 -> Bus Creator3/9  "Shutdown_Error"
  CanRx2/2 -> Bus Creator3/5  "Rear_Right_Wheel_Speed"
  CanRx2/3 -> Bus Creator3/6  "Rear_Wheel_Speed"
  CanRx5/1 -> Bus Creator3/7  "Steering_Angle"
  CanRx8/1 -> Bus Creator3/8  "Yaw"
  CanRx1/1 -> Bus Creator3/1  "Front_Left_Wheel_Speed"
  CanRx1/2 -> Bus Creator3/2  "Front_Right_Wheel_Speed"
  CanRx2/1 -> Bus Creator3/4  "Rear_Left_Wheel_Speed"
  Bus Creator3/1 -> Sensor_Data/1  "Sensor_Data"
  CanRx1/3 -> Bus Creator3/3  "Vehicle_Speed"

== system TBRe19_ECU_SequentialTests/TSS/Comms_And_Data_Output_Layer/Hardwired_Ouputs ==
  note: Turns the MCU on
  PostPL_Data : Inport
  AnalogOutput2 : S-Function  Description=This block interface the 8 Analog Outputs. The analog outputs are 0/20V. Voltage input is set in mV  FunctionName=NsiIo_AnalogOutput  Parameters=Channel,Feedback  SFunctionDeploymentMode=off  EnableBusSupport=off  mask(MUXlink I/O Analog Output){Channel=1, Feedback=off, RANGE=0 / 20 Volts}
      mask prompts: Channel "Channel ?"; Feedback "Read Back Analog out"; RANGE "Voltage Range"
      mask help: This block interface the 8 Analog Outputs. Channels 1 to 4 are 0/10V, and the channels 5 to 8 are0/20V. Voltage input is set in mV
      mask init:
      | NsiIo_AnalogOutput_InitializationFcn();
      settings: OpenFcn=NsiIo_AnalogOutput_OpenFcn();
      mask Help:
      | eval('block=get_param(gcb, ''RTWdata'');')
      | web([docroot '\toolbox\MUXlink\html\blocks/' block.MUXlink_BlockType '.html'])
      mask Callback Channel: NsiIo_AnalogOutput_ApplyFcn(1);
      mask Display: image(imread('nsi.bmp'));text(0.5, 0.2, 'AnalogOutput_1\n\n0 / 20 Volts', 'horizontalAlignment', 'center', 'verticalAlignment', 'base');plot([0.05 0.05 0.05 0.05 0.05 0.05 0.05 0.05 0.05 0.05]);port_label('input', 1, 'E3');
  Bus Selector : BusSelector  OutputSignals=Hardwired_Peripherals.TSS
  wires:
  PostPL_Data/1 -> Bus Selector/1
  Bus Selector/1 -> AnalogOutput2/1  "<TSS>"

== system TBRe19_ECU_SequentialTests/TSS/Post_Processing_Layer/Hardwired_Peripherals ==
  note: Talk to Wilkins about when you want pump and fans
      | power switching between Vicor and LV to occur
  note: Set TSS to 8V when it is true (this turns on a MOSFET)
  VFL_Data : Inport
  8V : Constant  Value=8000  OutDataTypeStr=Inherit: Inherit via back propagation
  Bus Creator : BusCreator  Inputs=7
  Bus Selector3 : BusSelector  OutputSignals=VOM_Data.TSS
  Ground : Constant  Value=0  OutDataTypeStr=Inherit: Inherit via back propagation
  Switch4 : Switch  Criteria=u2 > Threshold  OutDataTypeStr=uint16
  Hardwired_Peripherals : Outport
  wires:
  VFL_Data/1 -> Bus Selector3/1
  Bus Creator/1 -> Hardwired_Peripherals/1  "Hardwired_Peripherals"
  Switch4/1 -> Bus Creator/3  "TSS"
  Ground/1 -> Switch4/3
  Bus Selector3/1 -> Switch4/2  "<TSS>"
  8V/1 -> Switch4/1

== system TBRe19_ECU_SequentialTests/TSS/Vehicle_Functionality_Layer/Vehicle_Operation_Mode ==
  PrePL_Data : Inport
  Bus Creator : BusCreator  Inputs=5
  TSS : Subsystem
  VOM_Data : Outport
  wires:
  Bus Creator/1 -> VOM_Data/1  "Vehicle_Operation_Data"
  PrePL_Data/1 -> TSS/1(PrePL_Data)
  TSS/1(TS_StartUp) -> Bus Creator/5  "TSS"

== system TBRe19_ECU_SequentialTests/TSSBrake/Comms_And_Data_Acquisition_Layer/BMS_CAN ==
  note: Overall Functionality:
      | Read CAN messages related to BMS
  Bus Creator4 : BusCreator  Inputs=9
  CanRx6 : S-Function  FunctionName=NsiCan_Rx_Ext  Parameters=data_can,channel,msg_name,ident,ident_type,dlc,signals,is_trigger,is_physical,is_canfd,is_rxgw  SFunctionDeploymentMode=off  EnableBusSupport=off  mask(MUXlink Can Rx){data_can=1;HIGH_SPEED;500Kbps;120 Ohm;C:\Users\TBRe-admin\Documents\Database\TBRe19_DBC_190517.dbc;0;;;0;HIGH_SPEED;500Kbps;120 Ohm;C:\Users\TBRe-admin\Documents\Database\TBRe19_DBC_190517.dbc;0;;;0;HIGH_SPEED;1000Kbps;120 Ohm;D:\TOOLS\MUXLINK\R2011b\MUXlink\misc\BASE_CAN_MUXLAB4.dbc;0;;;0;HIGH_SPEED;500Kbps;120 Ohm;D:\TOOLS\MUXLINK\R2011b\MUXlink\misc\j1939_adapt.dbc;0;;;0;HIGH_SPEED;1000Kbps;No;D:\TOOLS\MUXLINK\R2011b\MUXlink\misc\BASE_CAN_MUXLAB4.dbc;0;;, channel=1, msg_name=BMS_Feedback_1, ident=0x050, ident_type=STD, dlc=7, signals=Instant_Pack_Voltage;1;0;16;1.000000;0.000000;_;Pack_SOC;1;16;16;1.000000;0.000000;_;Pack_Current;1;32;-16;1.000000;64.000000;_;Acc_Fan_Speed;1;48;8;1.000000;0.000000;_, is_trigger=0, is_physical=0, is_canfd=0, is_rxgw=0}
      mask prompts: data_can "data can"; msg_name "msg name"
      mask help: Receive a frame from a CAN channel.
      mask init:
      | NsiCan_Rx_Ext_InitializationFcn();
      settings: OpenFcn=NsiCan_Rx_Ext_OpenFcn();
      mask Help:
      | eval('block=get_param(gcb, ''RTWdata'');')
      | web([docroot '\toolbox\MUXlink\html\blocks/' block.MUXlink_BlockType '.html'])
      mask Callback data_can: NsiCan_Rx_Ext_ApplyFcn(1);
      mask Callback channel: NsiCan_Rx_Ext_ApplyFcn(2);
      mask Callback msg_name: NsiCan_Rx_Ext_ApplyFcn(3);
      mask Callback ident: NsiCan_Rx_Ext_ApplyFcn(4);
      mask Callback ident_type: NsiCan_Rx_Ext_ApplyFcn(5);
      mask Callback dlc: NsiCan_Rx_Ext_ApplyFcn(6);
      mask Callback signals: NsiCan_Rx_Ext_ApplyFcn(7);
      mask Callback is_trigger: NsiCan_Rx_Ext_ApplyFcn(8);
      mask Callback is_physical: NsiCan_Rx_Ext_ApplyFcn(9);
      mask Callback is_canfd: NsiCan_Rx_Ext_ApplyFcn(10);
      mask Callback is_rxgw: NsiCan_Rx_Ext_ApplyFcn(11);
      mask Display: image(imread('nsi.bmp'));text(0.5, 0.3, 'RX_BMS_Feedback_1_CAN1', 'horizontalAlignment', 'center', 'verticalAlignment', 'base');plot([0.05 0.05 0.05 0.05 0.05 0.05 0.05 0.05 0.05 0.05]); port_label('output',1, 'Instant_Pack_Voltage'); port_label('output',2, 'Pack_SOC'); port_label('output',3, 'Pack_Current'); port_label('output',4, 'Acc_Fan_Speed'); port_label('output',5, 'Status');
  CanRx7 : S-Function  FunctionName=NsiCan_Rx_Ext  Parameters=data_can,channel,msg_name,ident,ident_type,dlc,signals,is_trigger,is_physical,is_canfd,is_rxgw  SFunctionDeploymentMode=off  EnableBusSupport=off  mask(MUXlink Can Rx){data_can=1;HIGH_SPEED;500Kbps;No;C:\Users\uvind\OneDrive\Programming\Team Bath Racing Electric\TBRe19_DBC_190621.dbc;0;;;0;HIGH_SPEED;500Kbps;120 Ohm;C:\Users\TBRe-admin\Documents\Database\TBRe19_DBC_190517.dbc;0;;;0;HIGH_SPEED;1000Kbps;120 Ohm;D:\TOOLS\MUXLINK\R2011b\MUXlink\misc\BASE_CAN_MUXLAB4.dbc;0;;;0;HIGH_SPEED;500Kbps;120 Ohm;D:\TOOLS\MUXLINK\R2011b\MUXlink\misc\j1939_adapt.dbc;0;;;0;HIGH_SPEED;1000Kbps;No;D:\TOOLS\MUXLINK\R2011b\MUXlink\misc\BASE_CAN_MUXLAB4.dbc;0;;, channel=1, msg_name=BMS_Feedback_2, ident=0x051, ident_type=STD, dlc=8, signals=Avg_Cell_Voltage;1;32;16;1.000000;0.000000;_;High_Cell_Voltage;1;16;16;1.000000;0.000000;_;High_Cell_ID;1;56;8;1.000000;0.000000;_;Low_Cell_Voltage;1;0;16;1.000000;0.000000;_;Low_Cell_ID;1;48;8;1.000000;0.000000;_, is_trigger=0, is_physical=0, is_canfd=0, is_rxgw=0}
      mask prompts: data_can "data can"; msg_name "msg name"
      mask help: Receive a frame from a CAN channel.
      mask init:
      | NsiCan_Rx_Ext_InitializationFcn();
      settings: OpenFcn=NsiCan_Rx_Ext_OpenFcn();
      mask Help:
      | eval('block=get_param(gcb, ''RTWdata'');')
      | web([docroot '\toolbox\MUXlink\html\blocks/' block.MUXlink_BlockType '.html'])
      mask Callback data_can: NsiCan_Rx_Ext_ApplyFcn(1);
      mask Callback channel: NsiCan_Rx_Ext_ApplyFcn(2);
      mask Callback msg_name: NsiCan_Rx_Ext_ApplyFcn(3);
      mask Callback ident: NsiCan_Rx_Ext_ApplyFcn(4);
      mask Callback ident_type: NsiCan_Rx_Ext_ApplyFcn(5);
      mask Callback dlc: NsiCan_Rx_Ext_ApplyFcn(6);
      mask Callback signals: NsiCan_Rx_Ext_ApplyFcn(7);
      mask Callback is_trigger: NsiCan_Rx_Ext_ApplyFcn(8);
      mask Callback is_physical: NsiCan_Rx_Ext_ApplyFcn(9);
      mask Callback is_canfd: NsiCan_Rx_Ext_ApplyFcn(10);
      mask Callback is_rxgw: NsiCan_Rx_Ext_ApplyFcn(11);
      mask Display: image(imread('nsi.bmp'));text(0.5, 0.3, 'RX_BMS_Feedback_2_CAN1', 'horizontalAlignment', 'center', 'verticalAlignment', 'base');plot([0.05 0.05 0.05 0.05 0.05 0.05 0.05 0.05 0.05 0.05]); port_label('output',1, 'Avg_Cell_Voltage'); port_label('output',2, 'High_Cell_Voltage'); port_label('output',3, 'High_Cell_ID'); port_label('output',4, 'Low_Cell_Voltage'); port_label('output',5, 'Low_Cell_ID'); port_label('output',6, 'Status');
  BMS_Data : Outport
  wires:
  CanRx6/5 -> ?
  CanRx7/6 -> ?
  CanRx6/3 -> Bus Creator4/3  "Pack_Current"
  CanRx6/1 -> Bus Creator4/1  "Instant_Pack_Voltage"
  CanRx7/3 -> Bus Creator4/7  "High_Cell_ID"
  CanRx6/4 -> Bus Creator4/4  "Acc_Fan_Speed"
  CanRx7/1 -> Bus Creator4/5  "Abg_Cell_Voltage"
  Bus Creator4/1 -> BMS_Data/1  "BMS_Data"
  CanRx7/5 -> Bus Creator4/9  "Low_Cell_ID"
  CanRx7/2 -> Bus Creator4/6  "High_Cell_Voltage"
  CanRx7/4 -> Bus Creator4/8  "Low_Cell_Voltage"
  CanRx6/2 -> Bus Creator4/2  "Pack_SOC"

== system TBRe19_ECU_SequentialTests/TSSBrake/Comms_And_Data_Acquisition_Layer/Hardwired_Inputs_2019 ==
  note: Action:
      | Put the inputs into bus and generate output
  note: Overall Functionality:
      | Get inputs from the physical input pins
  AIRs : Subsystem
  BMS : Subsystem
  Bus Creator : BusCreator  Inputs=18
  Buttons : Subsystem
  FrequentialInput1 : S-Function  FunctionName=NsiIo_FrequencyInput  Parameters=channel,max_freq,is_digital_input,DutyCycle,MUXlabType  SFunctionDeploymentMode=off  EnableBusSupport=off  mask(MUXlink I/O Frequential Input){channel=3, max_freq=10KHZ, is_digital_input=off, DutyCycle=off, MUXlabType=0}
      mask prompts: max_freq "Max Frequency"; is_digital_input "Used as Digital Input"; DutyCycle "Duty Cycle"; MUXlabType "MUXlab Type"
      mask help: Read Frequency from I/O Frequential Input.
      mask init:
      | NsiIo_FrequencyInput_InitializationFcn();
      settings: OpenFcn=NsiIo_FrequencyInput_OpenFcn();
      mask Help:
      | eval('block=get_param(gcb, ''RTWdata'');')
      | web([docroot '\toolbox\MUXlink\html\blocks/' block.MUXlink_BlockType '.html'])
      mask Callback channel: NsiIo_FrequencyInput_ApplyFcn(1);
      mask TypeOptions max_freq: 10KHZ | 100KHZ
      mask Callback max_freq: NsiIo_FrequencyInput_ApplyFcn(2);
      mask Callback is_digital_input: NsiIo_FrequencyInput_ApplyFcn(3);
      mask Callback DutyCycle: NsiIo_FrequencyInput_ApplyFcn(4);
      mask Display: image(imread('nsi.bmp'));text(0.5, 0.2, 'FrequencyInput_3  10KHZ', 'horizontalAlignment', 'center', 'verticalAlignment', 'base');plot([0.05 0.05 0.05 0.05 0.05 0.05 0.05 0.05 0.05 0.05]);port_label('output', 1, 'Freq C3');
  Pedal_Box : Subsystem
  VBat : S-Function  FunctionName=NsiIo_Vbat  SFunctionDeploymentMode=off  EnableBusSupport=off  mask(MUXlink I/O VBat){}
      mask help: Battery Voltage
      mask init:
      | NsiIo_Vbat_InitializationFcn();
      settings: OpenFcn=NsiIo_Vbat_OpenFcn();
      mask Help:
      | eval('block=get_param(gcb, ''RTWdata'');')
      | web([docroot '\toolbox\MUXlink\html\blocks/' block.MUXlink_BlockType '.html'])
      mask Display: image(imread('nsi.bmp'));text(0.5, 0.2, 'I/O VBat', 'horizontalAlignment', 'center', 'verticalAlignment', 'base');plot([0.05 0.05 0.05 0.05 0.05 0.05 0.05 0.05 0.05 0.05]);port_label('output', 1, 'Voltage');
  Hardwired_Inputs : Outport
  wires:
  VBat/1 -> Bus Creator/12  "LV_Battery_Voltage"
  FrequentialInput1/1 -> Bus Creator/13  "Fan_Freq"
  Bus Creator/1 -> Hardwired_Inputs/1
  Pedal_Box/1(Throttle1_Voltage) -> Bus Creator/1
  Pedal_Box/2(Throttle2_Voltage) -> Bus Creator/2
  Pedal_Box/3(Brake_Voltage) -> Bus Creator/3
  Buttons/1(btnRTD_Input) -> Bus Creator/6
  Buttons/2(btnX_Input) -> Bus Creator/7
  Buttons/3(btnY_Input) -> Bus Creator/8
  AIRs/1(AIRLow) -> Bus Creator/14
  AIRs/2(AIRHigh) -> Bus Creator/15
  Pedal_Box/4(Brake1_Pressure) -> Bus Creator/4
  Pedal_Box/5(Brake2_Pressure) -> Bus Creator/5
  Buttons/4(btnZ_Input) -> Bus Creator/9
  Buttons/5(btnPumpFan_Input) -> Bus Creator/10
  Buttons/6(btnAccyFan_Input) -> Bus Creator/11
  BMS/1(BMS_Multi1) -> Bus Creator/16
  BMS/2(BMS_Multi2) -> Bus Creator/17
  BMS/3(BMS_ChargeEnable) -> Bus Creator/18
